simulink model "sampleModel1713"  (R2023a)
settings: Solver=VariableStepAuto  StartTime=0.0  StopTime=10.0  RelTol=1e-3
libraries: hdlsllib x7, simulink x6
settings Model: Creator=user1  LastModifiedBy=user1

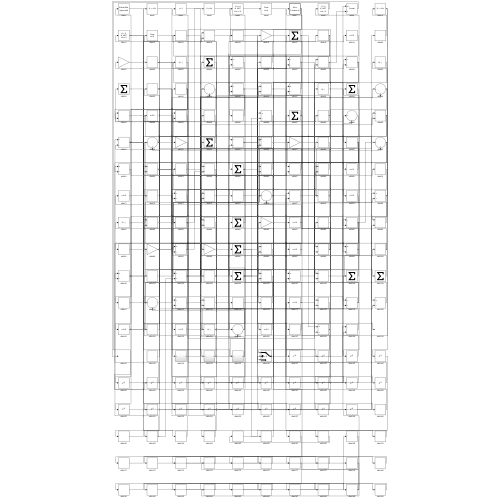
[thumbnail: Simulink's stored preview of the top-level diagram]
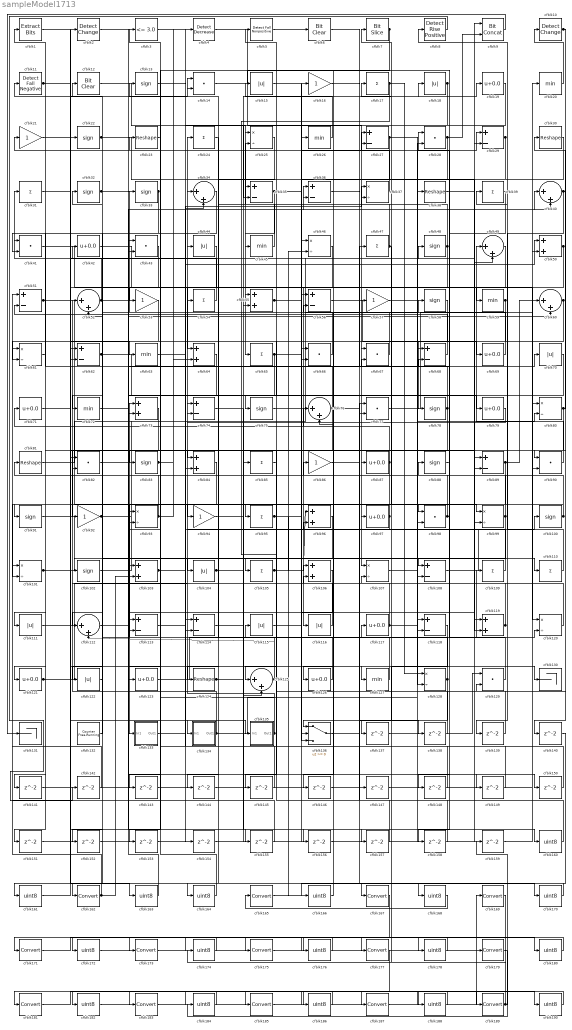
== system sampleModel1713 ==
  cfblk1 : simulink/Logic and Bit Operations/Extract Bits  bitsToExtract=Upper half  numBits=8  bitIdxRange=[0 7]  outScalingMode=Preserve fixed-point scaling
      settings: LibrarySourceBlock=|
      | hdlsllib/Logic and Bit
      | Operations/Extract Bits
  cfblk10 : simulink/Logic and Bit Operations/Detect Change  vinit=0  OutDataTypeStr=boolean
      settings: LibrarySourceBlock=|
      | hdlsllib/Logic and Bit
      | Operations/Detect
      | Change
  cfblk{13,22,32..33,48,58,75,78,83,88,91,100,102} (13 alike) : Signum
  cfblk{25,37,46,61,80,93,99,101,107,120,128} (11 alike) : Product  Inputs=*/  RndMeth=Zero  SaturateOnIntegerOverflow=on
  cfblk{50,55,64,73,84,96,103,106,119} (9 alike) : Sum
  cfblk{15,18,44,70,104,111,115..116,122} (9 alike) : Abs  SaturateOnIntegerOverflow=off
  cfblk{17,24,31,39,47,54,65,85,95,105,109..110} (12 alike) : Sum  Inputs=+
  cfblk{27,29,35..36,51,56,62,68,74,89,108,113..114,118} (14 alike) : Sum  Inputs=+-
  cfblk11 : hdlsllib/Logic and Bit Operations/Detect Fall Negative  vinit=0  OutDataTypeStr=boolean
  cfblk{34,40,49,52,60,76,112,125} (8 alike) : Sum  Inputs=|++
  cfblk{19,42,69,71,79,87,97,117,121,123,126} (11 alike) : Bias  Bias=0.0  SaturateOnIntegerOverflow=off
  cfblk12 : simulink/Logic and Bit Operations/Bit Clear  iBit=0
      settings: LibrarySourceBlock=|
      | hdlsllib/Logic and Bit
      | Operations/Bit Clear
  cfblk{23,30,38,81,124} (5 alike) : Reshape
  cfblk{20,26,45,59,63,72,127} (7 alike) : MinMax
  cfblk{14,28,41,43,66..67,77,82,90,98,129} (11 alike) : DotProduct  OutDataTypeStr=Inherit: Inherit via internal rule
  cfblk130 : Terminator
  cfblk131 : Terminator
  cfblk132 : hdlsllib/Sources/Counter Free-Running  NumBits=16  tsamp=-1
  cfblk133 : Subsystem
      settings: LibrarySourceBlock=|
      | hdlsllib/Ports &
      | Subsystems/Subsystem
  cfblk134 : Subsystem
      settings: LibrarySourceBlock=|
      | hdlsllib/Ports &
      | Subsystems/Subsystem
  cfblk135 : Subsystem
      settings: LibrarySourceBlock=|
      | hdlsllib/Ports &
      | Subsystems/Subsystem
  cfblk136 : Switch  SaturateOnIntegerOverflow=off  InputSameDT=off
  cfblk{137..159} (23 alike) : Delay  SampleTime=1
  cfblk{16,21,53,57,86,92,94} (7 alike) : Gain
  cfblk{160..161,163..164,166,168,170,172,174,176,178,180,182,184,186,188,190} (17 alike) : DataTypeConversion  OutDataTypeStr=uint8  SaturateOnIntegerOverflow=off  RndMeth=Floor
  cfblk{162,165,167,169,171,173,175,177,179,181,183,185,187,189} (14 alike) : DataTypeConversion  SaturateOnIntegerOverflow=off  RndMeth=Floor
  cfblk2 : simulink/Logic and Bit Operations/Detect Change  vinit=0  OutDataTypeStr=boolean
      settings: LibrarySourceBlock=|
      | hdlsllib/Logic and Bit
      | Operations/Detect
      | Change
  cfblk3 : hdlsllib/Logic and Bit Operations/Compare To Constant  relop=<=  const=3.0  OutDataTypeStr=boolean
  cfblk4 : simulink/Logic and Bit Operations/Detect Decrease  vinit=0.0  OutDataTypeStr=boolean
      settings: LibrarySourceBlock=|
      | hdlsllib/Logic and Bit
      | Operations/Detect
      | Decrease
  cfblk5 : hdlsllib/Logic and Bit Operations/Detect Fall Nonpositive  vinit=0  OutDataTypeStr=boolean
  cfblk6 : simulink/Logic and Bit Operations/Bit Clear  iBit=0
      settings: LibrarySourceBlock=|
      | hdlsllib/Logic and Bit
      | Operations/Bit Clear
  cfblk7 : hdlsllib/Logic and Bit Operations/Bit Slice  lidx=7  ridx=0
  cfblk8 : hdlsllib/Logic and Bit Operations/Detect Rise Positive  vinit=0  OutDataTypeStr=boolean
  cfblk9 : hdlsllib/Logic and Bit Operations/Bit Concat  numInputs=2
  wires:
  cfblk54/1 -> cfblk21/1
  cfblk18/1 -> cfblk65/1, cfblk35/2
  cfblk101/1 -> cfblk105/1, cfblk48/1
  cfblk17/1 -> cfblk125/1, cfblk128/1
  cfblk135/1(Out1) -> cfblk24/1, cfblk23/1
  cfblk14/1 -> cfblk108/1
  cfblk58/1 -> cfblk107/1
  cfblk51/1 -> cfblk99/1, cfblk63/1, cfblk84/2
  cfblk126/1 -> cfblk73/1
  cfblk116/1 -> cfblk52/1
  cfblk117/1 -> cfblk34/1, cfblk120/2
  cfblk93/1 -> cfblk81/1, cfblk64/2
  cfblk48/1 -> cfblk116/1, cfblk13/1
  cfblk108/1 -> cfblk8/1
  cfblk90/1 -> cfblk49/1
  cfblk5/1 -> cfblk6/1
  cfblk76/1 -> cfblk41/1, cfblk145/1, cfblk150/1
  cfblk124/1 -> cfblk70/1, cfblk18/1
  cfblk66/1 -> cfblk32/1
  cfblk132/1 -> cfblk12/1
  cfblk69/1 -> cfblk33/1
  cfblk134/1(Out1) -> cfblk102/1, cfblk38/1
  cfblk33/1 -> cfblk111/1, cfblk112/1, cfblk41/2
  cfblk111/1 -> cfblk44/1
  cfblk82/1 -> cfblk9/1
  cfblk91/1 -> cfblk108/2
  cfblk44/1 -> cfblk72/1
  cfblk61/1 -> cfblk121/1
  cfblk12/1 -> cfblk25/1
  cfblk11/1 -> cfblk128/2, cfblk163/1
  cfblk41/1 -> cfblk120/1
  cfblk87/1 -> cfblk101/2, cfblk71/1
  cfblk20/1 -> cfblk10/1
  cfblk89/1 -> cfblk98/1, cfblk93/2, cfblk60/1
  cfblk67/1 -> cfblk3/1
  cfblk64/1 -> cfblk73/2
  cfblk7/1 -> cfblk126/1, cfblk83/1
  cfblk9/1 -> cfblk131/1
  cfblk75/1 -> cfblk58/1
  cfblk45/1 -> cfblk25/2
  cfblk4/1 -> cfblk67/1
  cfblk120/1 -> cfblk17/1
  cfblk105/1 -> cfblk96/1, cfblk46/2, cfblk119/2
  cfblk49/1 -> cfblk97/1
  cfblk74/1 -> cfblk125/2
  cfblk62/1 -> cfblk118/1, cfblk135/1(In1), cfblk60/2
  cfblk23/1 -> cfblk53/1
  cfblk59/1 -> cfblk75/1, cfblk78/1, cfblk61/2
  cfblk10/1 -> cfblk129/2, cfblk90/1
  cfblk30/1 -> cfblk98/2
  cfblk109/1 -> cfblk74/1
  cfblk99/1 -> cfblk104/1, cfblk7/1
  cfblk42/1 -> cfblk64/1
  cfblk65/1 -> cfblk127/1, cfblk143/1
  cfblk37/1 -> cfblk1/1
  cfblk71/1 -> cfblk134/1(In1)
  cfblk84/1 -> cfblk133/1(In1)
  cfblk92/1 -> cfblk47/1, cfblk67/2
  cfblk125/1 -> cfblk11/1, cfblk112/2
  cfblk113/1 -> cfblk50/1
  cfblk19/1 -> cfblk114/2
  cfblk104/1 -> cfblk106/1, cfblk14/1
  cfblk38/1 -> cfblk99/2
  cfblk68/1 -> cfblk51/2
  cfblk52/1 -> cfblk79/1, cfblk31/1
  cfblk55/1 -> cfblk26/1, cfblk27/2
  cfblk129/1 -> cfblk28/1
  cfblk15/1 -> cfblk66/2
  cfblk102/1 -> cfblk56/1
  cfblk128/1 -> cfblk54/1, cfblk146/1
  cfblk100/1 -> cfblk52/2, cfblk91/1
  cfblk26/1 -> cfblk15/1
  cfblk97/1 -> cfblk95/1, cfblk96/2
  cfblk46/1 -> cfblk55/1
  cfblk60/1 -> cfblk103/1, cfblk153/1
  cfblk47/1 -> cfblk36/1, cfblk87/1
  cfblk56/1 -> cfblk69/1
  cfblk110/1 -> cfblk39/1
  cfblk79/1 -> cfblk74/2
  cfblk80/1 -> cfblk92/1, cfblk30/1
  cfblk115/1 -> cfblk29/1
  cfblk72/1 -> cfblk110/1
  cfblk123/1 -> cfblk109/1
  cfblk81/1 -> cfblk19/1
  cfblk77/1 -> cfblk20/1
  cfblk95/1 -> cfblk16/1, cfblk166/1
  cfblk16/1 -> cfblk59/1
  cfblk133/1(Out1) -> cfblk100/1
  cfblk35/1 -> cfblk45/1, cfblk27/1
  cfblk83/1 -> cfblk123/1, cfblk4/1
  cfblk24/1 -> cfblk124/1
  cfblk50/1 -> cfblk57/1, cfblk62/2
  cfblk27/1 -> cfblk76/2, cfblk130/1
  cfblk107/1 -> cfblk80/2
  cfblk63/1 -> cfblk37/1
  cfblk121/1 -> cfblk34/2, cfblk14/2
  cfblk96/1 -> cfblk122/1
  cfblk21/1 -> cfblk22/1
  cfblk127/1 -> cfblk93/1
  cfblk114/1 -> cfblk85/1
  cfblk57/1 -> cfblk28/2
  cfblk98/1 -> cfblk37/2, cfblk68/2
  cfblk28/1 -> cfblk118/2, cfblk9/2
  cfblk1/1 -> cfblk82/1
  cfblk43/1 -> cfblk162/1
  cfblk103/1 -> cfblk36/2, cfblk40/2
  cfblk78/1 -> cfblk42/1, cfblk84/1
  cfblk32/1 -> cfblk89/2, cfblk94/1
  cfblk106/1 -> cfblk113/1
  cfblk29/1 -> cfblk136/1, cfblk136/3
  cfblk119/1 -> cfblk5/1, cfblk88/1
  cfblk40/1 -> cfblk139/1, cfblk140/1
  cfblk22/1 -> cfblk119/1, cfblk149/1
  cfblk85/1 -> cfblk35/1
  cfblk136/1 -> cfblk77/2
  cfblk112/1 -> cfblk40/1
  cfblk122/1 -> cfblk82/2
  cfblk118/1 -> cfblk137/1
  cfblk137/1 -> cfblk129/1
  cfblk36/1 -> cfblk138/1
  cfblk138/1 -> cfblk107/2
  cfblk139/1 -> cfblk62/1
  cfblk34/1 -> cfblk141/1
  cfblk141/1 -> cfblk89/1
  cfblk8/1 -> cfblk142/1
  cfblk142/1 -> cfblk101/1
  cfblk143/1 -> cfblk66/1
  cfblk25/1 -> cfblk144/1
  cfblk144/1 -> cfblk29/2
  cfblk145/1 -> cfblk114/1
  cfblk146/1 -> cfblk76/1
  cfblk6/1 -> cfblk147/1
  cfblk147/1 -> cfblk50/2
  cfblk88/1 -> cfblk148/1
  cfblk148/1 -> cfblk106/2
  cfblk149/1 -> cfblk113/2
  cfblk150/1 -> cfblk136/2
  cfblk73/1 -> cfblk151/1
  cfblk151/1 -> cfblk55/2
  cfblk53/1 -> cfblk152/1
  cfblk152/1 -> cfblk46/1
  cfblk153/1 -> cfblk68/1
  cfblk3/1 -> cfblk154/1
  cfblk154/1 -> cfblk80/1
  cfblk31/1 -> cfblk155/1
  cfblk155/1 -> cfblk51/1
  cfblk94/1 -> cfblk156/1
  cfblk156/1 -> cfblk49/2
  cfblk13/1 -> cfblk157/1
  cfblk157/1 -> cfblk77/1
  cfblk39/1 -> cfblk158/1
  cfblk158/1 -> cfblk56/2
  cfblk159/1 -> cfblk90/2
  cfblk2/1 -> cfblk160/1
  cfblk160/1 -> cfblk115/1
  cfblk140/1 -> cfblk161/1
  cfblk161/1 -> cfblk2/1
  cfblk162/1 -> cfblk61/1, cfblk103/2
  cfblk163/1 -> cfblk43/1
  cfblk70/1 -> cfblk164/1
  cfblk164/1 -> cfblk43/2
  cfblk166/1 -> cfblk86/1
  cfblk86/1 -> cfblk168/1
  cfblk168/1 -> cfblk165/1
  cfblk165/1 -> cfblk170/1
  cfblk170/1 -> cfblk167/1
  cfblk167/1 -> cfblk172/1
  cfblk172/1 -> cfblk169/1
  cfblk169/1 -> cfblk174/1
  cfblk174/1 -> cfblk171/1
  cfblk171/1 -> cfblk176/1
  cfblk176/1 -> cfblk173/1
  cfblk173/1 -> cfblk178/1
  cfblk178/1 -> cfblk175/1
  cfblk175/1 -> cfblk180/1
  cfblk180/1 -> cfblk177/1
  cfblk177/1 -> cfblk182/1
  cfblk182/1 -> cfblk179/1
  cfblk179/1 -> cfblk184/1
  cfblk184/1 -> cfblk181/1
  cfblk181/1 -> cfblk186/1
  cfblk186/1 -> cfblk183/1
  cfblk187/1 -> cfblk189/1
  cfblk183/1 -> cfblk188/1
  cfblk188/1 -> cfblk185/1
  cfblk189/1 -> cfblk159/1, cfblk117/1
  cfblk185/1 -> cfblk190/1
  cfblk190/1 -> cfblk187/1

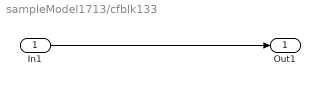
== system sampleModel1713/cfblk133 ==
  In1 : Inport
  Out1 : Outport
  wires:
  In1/1 -> Out1/1

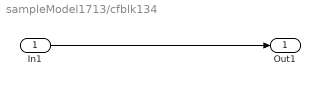
== system sampleModel1713/cfblk134 ==
  In1 : Inport
  Out1 : Outport
  wires:
  In1/1 -> Out1/1

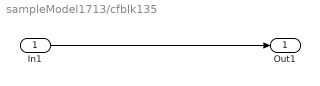
== system sampleModel1713/cfblk135 ==
  In1 : Inport
  Out1 : Outport
  wires:
  In1/1 -> Out1/1
